simulink model "lab3_2"  (R2020b)
settings: Solver=VariableStepAuto  StartTime=0.0  StopTime=10  MaxStep=0.01  RelTol=1e-3
InitFcn:
  | a0 = 2;
  | a1 = -5;
  | b0 = 5;
  | A = [0 1; -a0 -a1];
  | b = [0; b0];
  | 
  | am0 = 64;
  | am1 = 16;
  | Am = [0 1; -am0 -am1];
  | bm = [0; am0];
  | 
  | theta1 = (-am0 + a0)/b0;
  | theta2 = (-am1 + a1)/b0;
  | theta = [theta1; theta2];
  | kappa = b0/am0;
settings Model: Creator=Eeer12  LastModifiedBy=Eugene

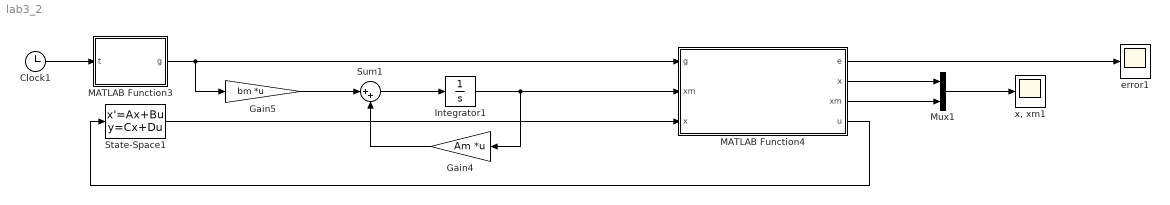
== system lab3_2 ==
  Clock1 : Clock
  Gain4 : Gain  Gain=Am  Multiplication=Matrix(K*u)
  Gain5 : Gain  Gain=bm  Multiplication=Matrix(K*u)
  Integrator1 : Integrator  InitialCondition=[0; 0]
  MATLAB Function3 : MATLAB Function  TreatAsAtomicUnit=on
  MATLAB Function4 : MATLAB Function  TreatAsAtomicUnit=on
  Mux1 : Mux  Inputs=2
  State-Space1 : StateSpace  A=A + [0 0; 20 20]  B=b  C=eye(2)  D=[0; 0]  InitialCondition=[0; 0]
  Sum1 : Sum  Inputs=|++
  error1 : Scope
  "x, xm1" : Scope
  wires:
  Clock1/1 -> MATLAB Function3/1(t)
  MATLAB Function3/1(g) -> Gain5/1, MATLAB Function4/1(g)
  Gain5/1 -> Sum1/1
  Sum1/1 -> Integrator1/1
  State-Space1/1 -> MATLAB Function4/3("x ")
  MATLAB Function4/4(u) -> State-Space1/1
  Integrator1/1 -> Gain4/1, MATLAB Function4/2("xm ")
  Gain4/1 -> Sum1/2
  MATLAB Function4/1(e) -> error1/1
  Mux1/1 -> "x, xm1"/1
  MATLAB Function4/2(x) -> Mux1/1
  MATLAB Function4/3(xm) -> Mux1/2

== matlab function lab3_2/MATLAB Function3 ==
  data: t input; g output
function g = fcn(t)

g = 10*cos(0.5*t) + 2*sin(t) + 12;

== matlab function lab3_2/MATLAB Function4 ==
  data: e output; x output; xm output; g input; xm input; x input; u output; kappa parameter; theta parameter
function [e, x, xm, u]  = fcn(g, xm, x, kappa, theta)

e = xm-x;
u = theta'*x + g/kappa;
